simulink model "platoon_project_string_stability4"  (Simulink 8.9)
settings: Solver=VariableStepAuto  StartTime=0.0  StopTime=50  FixedStep=0.1  RelTol=1e-3  EnableMultiTasking=on
values from neighbouring files (symbols this model uses):
  k1 = 1.3244    [platoon_stability.m]    (also in platoon_stability_ed.m = 0.0244)
  k2 = -1.2211    [platoon_stability.m]    (also in platoon_stability_ed.m = -1.7211)
  q = 0.1    [platoon_stability.m]    (also in platoon_stability_ed.m = 0.2)
  tau = 1.34    [platoon_stability.m]    (also in platoon_stability_ed.m = 1.24)
  tnet_table = [57.5127074443 119.897368421 182.282029398 223.675296349 261.549751738 274.206057597 279.305263158 283.689473684 288.073684211 292.467532318 296.875779086 301.284025854 ... (400 elements, 20x20)]    [enginemap.mat]    (also in genmap.m = griddata(map_ford(:,1), map_ford(:,4), map_ford(:,2), we_tab)
  we_max = 471.2    [enginemap.mat]    (also in genmap.m = max(map_ford(:,1)))
  we_min = 57.6    [enginemap.mat]    (also in genmap.m = min(map_ford(:,1)))
undefined symbols (not defined in the file or in its folder): c_aero, delay_brake, F_roll, h, I_e, I_wheel, KB, mass, max_throttle, max_throttle_rate, min_throttle, mu_B, mu_C, mu_D, mu_E, P_po, Rdrive, sigbuilder_block, tau_brake, tau_throttle, throttle_o, w_wheel_o, we_o, x_dot_o
libraries: simulink x8
(part 3 of 3)

== system platoon_project_string_stability4/4th Vehicle/Wheel Dynamics/Right Front Wheel/Tire Model ==
  note: rw-v
  note: Magic Tire Formula
  note: Slip ratio
  note: divide by 0를 없애기 위해
      | Switch Block을 사용했다
  Wheel Speed : Inport
  Vehicle Speed : Inport  Port=2
  Constant : Constant  Value=0.01
  Constant1 : Constant  Value=0.01
  Fcn : Fcn  Expr=mu_D*sin(mu_C*atan(mu_B*u-mu_E*(mu_B*u-atan(mu_B*u))))
  Gain : Gain  SaturateOnIntegerOverflow=on  OutDataTypeStr=Inherit: Same as input  ParamDataTypeStr=Inherit: Same as input
  Product : Product  Inputs=/*  SaturateOnIntegerOverflow=on  RndMeth=Zero  InputSameDT=on  OutDataTypeStr=Inherit: Same as first input
  Product1 : Product  Inputs=*/  SaturateOnIntegerOverflow=on  RndMeth=Zero  InputSameDT=on  OutDataTypeStr=Inherit: Same as first input
  Sum1 : Sum  Inputs=+-  SaturateOnIntegerOverflow=on  InputSameDT=on  OutDataTypeStr=Inherit: Same as first input
  Switch : Switch  SaturateOnIntegerOverflow=on  InputSameDT=on
  Switch1 : Switch  Threshold=0.01  SaturateOnIntegerOverflow=on  InputSameDT=on
  Switch2 : Switch  Threshold=0.01  SaturateOnIntegerOverflow=on  InputSameDT=on
  wheel radius1 : Gain  Gain=h  SaturateOnIntegerOverflow=on  OutDataTypeStr=Inherit: Same as input  ParamDataTypeStr=Inherit: Same as input
  Tractive Force : Outport
  RF_slip : Outport  Port=2
  wires:
  wheel radius1/1 -> Sum1/1, Switch1/1, Switch1/2
  Sum1/1 -> Switch/2, Product/2, Product1/1
  Product/1 -> Switch/1
  Product1/1 -> Switch/3
  Switch/1 -> Gain/1, RF_slip/1  "slip"
  Wheel Speed/1 -> wheel radius1/1
  Fcn/1 -> Tractive Force/1
  Vehicle Speed/1 -> Sum1/2, Switch2/1, Switch2/2
  Gain/1 -> Fcn/1
  Constant/1 -> Switch1/3
  Switch1/1 -> Product/1
  Switch2/1 -> Product1/2
  Constant1/1 -> Switch2/3

== system platoon_project_string_stability4/4th Vehicle/Wheel Dynamics/Right Rear Wheel/Tire Model ==
  Wheel Speed : Inport
  Vehicle Speed : Inport  Port=2
  Constant : Constant  Value=0.01
  Constant1 : Constant  Value=0.01
  Fcn : Fcn  Expr=mu_D*sin(mu_C*atan(mu_B*u-mu_E*(mu_B*u-atan(mu_B*u))))
  Gain : Gain  SaturateOnIntegerOverflow=on  OutDataTypeStr=Inherit: Same as input  ParamDataTypeStr=Inherit: Same as input
  Product : Product  Inputs=/*  SaturateOnIntegerOverflow=on  RndMeth=Zero  InputSameDT=on  OutDataTypeStr=Inherit: Same as first input
  Product1 : Product  Inputs=*/  SaturateOnIntegerOverflow=on  RndMeth=Zero  InputSameDT=on  OutDataTypeStr=Inherit: Same as first input
  Sum1 : Sum  Inputs=+-  SaturateOnIntegerOverflow=on  InputSameDT=on  OutDataTypeStr=Inherit: Same as first input
  Switch : Switch  SaturateOnIntegerOverflow=on  InputSameDT=on
  Switch1 : Switch  Threshold=0.01  SaturateOnIntegerOverflow=on  InputSameDT=on
  Switch2 : Switch  Threshold=0.01  SaturateOnIntegerOverflow=on  InputSameDT=on
  wheel radius1 : Gain  Gain=h  SaturateOnIntegerOverflow=on  OutDataTypeStr=Inherit: Same as input  ParamDataTypeStr=Inherit: Same as input
  Tractive Force : Outport
  RR_slip : Outport  Port=2
  wires:
  wheel radius1/1 -> Sum1/1, Switch1/1, Switch1/2
  Sum1/1 -> Switch/2, Product/2, Product1/1
  Product/1 -> Switch/1
  Product1/1 -> Switch/3
  Switch/1 -> Gain/1, RR_slip/1  "slip"
  Wheel Speed/1 -> wheel radius1/1
  Fcn/1 -> Tractive Force/1
  Vehicle Speed/1 -> Sum1/2, Switch2/1, Switch2/2
  Gain/1 -> Fcn/1
  Constant/1 -> Switch1/3
  Switch1/1 -> Product/1
  Switch2/1 -> Product1/2
  Constant1/1 -> Switch2/3

== matlab function                ACC Based On DIstance             ==
  data: L input double; ai input double; Throttle_Angle_err output double; Pmc_err output double; dist_gap input double
function [Throttle_Angle_err, Pmc_err] = converter(L, ai, dist_gap)

Throttle_Angle_err = 0;
Pmc_err = 0;


if ai > 0 && dist_gap > L
    Throttle_Angle_err =  0.75;
    Pmc_err = 0;
elseif ai > 0 && dist_gap < L
    Throttle_Angle_err =  1;
    Pmc_err =  0;
elseif ai < 0 && dist_gap > L
    Throttle_Angle_err =  0;
    Pmc_err =  0.75;
elseif ai < 0 && dist_gap < L
    Throttle_Angle_err =  0;
    Pmc_err =  1;
end

end

== matlab function                ACC Based On DIstance            ==
  data: L input double; ai input double; Throttle_Angle_err output double; Pmc_err output double; dist_gap input double
function [Throttle_Angle_err, Pmc_err] = converter(L, ai, dist_gap)

Throttle_Angle_err = 0;
Pmc_err = 0;


if ai > 0 && dist_gap > L
    Throttle_Angle_err =  0.75;
    Pmc_err = 0;
elseif ai > 0 && dist_gap < L
    Throttle_Angle_err =  1;
    Pmc_err =  0;
elseif ai < 0 && dist_gap > L
    Throttle_Angle_err =  0;
    Pmc_err =  0.75;
elseif ai < 0 && dist_gap < L
    Throttle_Angle_err =  0;
    Pmc_err =  1;
end

end

== matlab function                ACC Based On DIstance               ==
  data: L input double; ai input double; Throttle_Angle_err output double; Pmc_err output double; dist_gap input double
function [Throttle_Angle_err, Pmc_err] = converter(L, ai, dist_gap)

Throttle_Angle_err = 0;
Pmc_err = 0;


if ai > 0 && dist_gap > L
    Throttle_Angle_err =  0.75;
    Pmc_err = 0;
elseif ai > 0 && dist_gap < L
    Throttle_Angle_err =  1;
    Pmc_err =  0;
elseif ai < 0 && dist_gap > L
    Throttle_Angle_err =  0;
    Pmc_err =  0.75;
elseif ai < 0 && dist_gap < L
    Throttle_Angle_err =  0;
    Pmc_err =  1;
end

end

== matlab function                ACC Based On DIstance              ==
  data: L input double; ai input double; Throttle_Angle_err output double; Pmc_err output double; dist_gap input double
function [Throttle_Angle_err, Pmc_err] = converter(L, ai, dist_gap)

Throttle_Angle_err = 0;
Pmc_err = 0;


if ai > 0 && dist_gap > L
    Throttle_Angle_err =  0.75;
    Pmc_err = 0;
elseif ai > 0 && dist_gap < L
    Throttle_Angle_err =  1;
    Pmc_err =  0;
elseif ai < 0 && dist_gap > L
    Throttle_Angle_err =  0;
    Pmc_err =  0.75;
elseif ai < 0 && dist_gap < L
    Throttle_Angle_err =  0;
    Pmc_err =  1;
end

end
